simulink model "verify_PV_Generator_mdl"  (R2018b)
settings: Solver=ode45  StartTime=0  StopTime=365*24*3600  RelTol=1e-3  EnableMultiTasking=on
InitFcn:
  | load('DE_TRY2010_13_averageYear')
undefined symbols (not defined in the file or in its folder): path_carnot
libraries: carnot x3
settings Model: Creator=drhf  LastModifiedBy=drhf
settings DataIOCC: SaveFormat=Array  SignalLoggingSaveFormat=ModelDataLogs
settings OptimizationCC: ExpressionDepthLimit=2147483647  LifeSpan=inf
settings DebuggingCC: UnderspecifiedInitializationDetection=Classic  MergeDetectMultiDrivingBlocksExec=none  SolverPrmCheckMsg=warning  FcnCallInpInsideContextMsg=warning  StateNameClashWarn=warning  SFUnexpectedBacktrackingDiag=warning  SFNoUnconditionalDefaultTransitionDiag=warning  SFExecutionAtInitializationDiag=none
settings HardwareCC: ProdBitPerPointer=32  ProdBitPerSizeT=32  ProdBitPerPtrDiffT=32  ProdLargestAtomicFloat=None  ProdIntDivRoundTo=Undefined  ProdEndianess=Unspecified  ProdWordSize=32  ProdHWDeviceType=32-bit Generic
settings ModelReferenceCC: PropagateSignalLabelsOutOfModel=off
settings SFSimCC: SimUseLocalCustomCode=off
settings RTWCC: RTWUseLocalCustomCode=off
settings CodeAppCC: StateflowObjectComments=on
settings GRTTargetCC: TargetLangStandard=C89/C90 (ANSI)  GeneratePreprocessorConditionals=Disable all  CombineOutputUpdateFcns=off  GRTInterface=on
settings ConfigComp: CovMetricSettings=dw  CovHtmlReporting=on  CovSaveCumulativeToWorkspaceVar=on  CovSaveSingleToWorkspaceVar=on  CovExternalEMLEnable=off

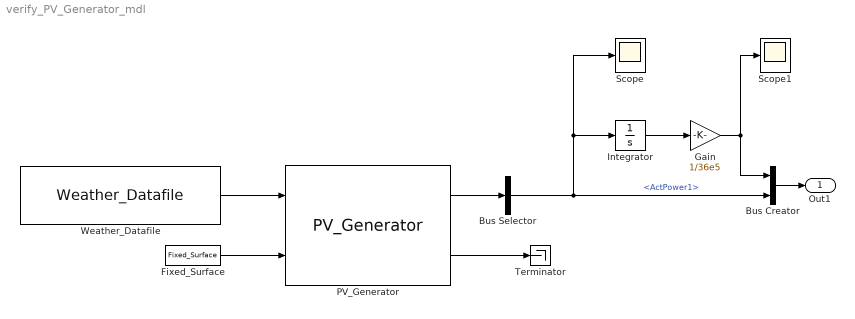
== system verify_PV_Generator_mdl ==
  Bus Creator : BusCreator  Inputs=2
  Bus Selector : BusSelector  OutputSignals=ActPower1
  Fixed_Surface : carnot/Weather/Fixed_Surface  colangle=30  colazi=0  colrot=0
      settings: SourceProductName=Carnot
  Gain : Gain  Gain=1/36e5
  Integrator : Integrator
  PV_Generator : carnot/Source/Electric_Generator/PV_Generator  Wp=1000  delta_Wp_K=0.0047  fgen=0.91 % 0.06 power missmatch, 0.01 diodes, 0.02 data sheet tolerance
      settings: SourceProductName=Carnot
  Scope : Scope
  Scope1 : Scope
  Terminator : Terminator
  Weather_Datafile : carnot/Weather/Weather_Datafile  PathName=path_carnot('data')  FileName='DE_TRY2010_13_averageYear.mat'  UserParam=off  VariableName=DE_TRY2010_13_averageYear  SampleTime=3600
      settings: SourceProductName=Carnot
  Out1 : Outport
  wires:
  PV_Generator/1 -> Bus Selector/1
  PV_Generator/2 -> Terminator/1
  Fixed_Surface/1 -> PV_Generator/2
  Integrator/1 -> Gain/1
  Gain/1 -> Bus Creator/1, Scope1/1
  Bus Creator/1 -> Out1/1
  Weather_Datafile/1 -> PV_Generator/1
  Bus Selector/1 -> Bus Creator/2, Integrator/1, Scope/1  "<ActPower1>"
